simulink model "prob1"  (R2020b)
settings: Solver=VariableStepAuto  StartTime=0.0  StopTime=10.0  RelTol=1e-3
undefined symbols (not defined in the file): b, k1, k12, M1, M2
settings Model: Creator=nadee  LastModifiedBy=nadee

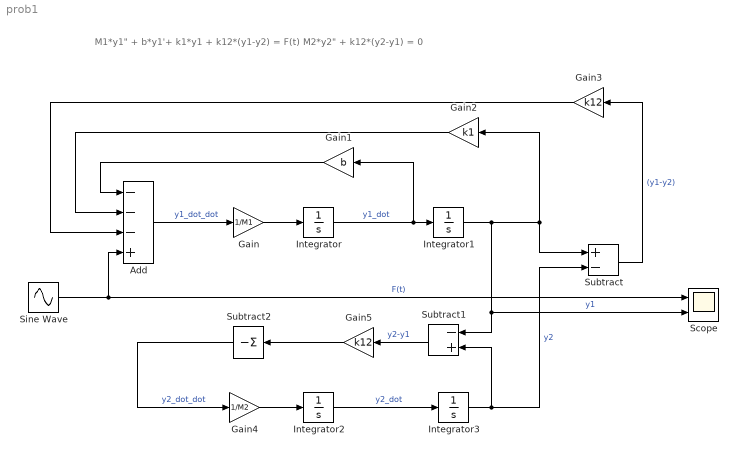
== system prob1 ==
  note: M1*y1" + b*y1'+ k1*y1 + k12*(y1-y2) = F(t)
      | M2*y2" + k12*(y2-y1) = 0
  Add : Sum  Inputs=---+
  Gain : Gain  Gain=1/M1
  Gain1 : Gain  Gain=b
  Gain2 : Gain  Gain=k1
  Gain3 : Gain  Gain=k12
  Gain4 : Gain  Gain=1/M2
  Gain5 : Gain  Gain=k12
  Integrator{,1..3} (4 alike) : Integrator
  Scope : Scope  NumInputPorts=2
  Sine Wave : Sin  SampleTime=0
  Subtract : Sum  Inputs=+-
  Subtract1 : Sum  Inputs=-+
  Subtract2 : Sum  Inputs=-
  wires:
  Integrator/1 -> Integrator1/1, Gain1/1  "y1_dot"
  Integrator1/1 -> Subtract1/1, Scope/2, Gain2/1, Subtract/1  "y1"
  Add/1 -> Gain/1  "y1_dot_dot"
  Gain4/1 -> Integrator2/1
  Integrator2/1 -> Integrator3/1  "y2_dot"
  Integrator3/1 -> Subtract1/2, Subtract/2  "y2"
  Gain/1 -> Integrator/1
  Subtract/1 -> Gain3/1  "(y1-y2)"
  Gain1/1 -> Add/1
  Gain2/1 -> Add/2
  Gain3/1 -> Add/3
  Sine Wave/1 -> Scope/1, Add/4  "F(t)"
  Subtract1/1 -> Gain5/1  "y2-y1"
  Gain5/1 -> Subtract2/1
  Subtract2/1 -> Gain4/1  "y2_dot_dot"
